simulink model "Parameter_Estimation_2020b"  (R2021a)
settings: Solver=ode2  StartTime=0.0  StopTime=9.999  FixedStep=0.001  RelTol=1e-3  EnableMultiTasking=on
StopFcn:
  | clc;
  | display('--------------------------------------------')
  | display('Running Least Squares Estimatation')
  | display('--------------------------------------------')
  | 
  | L = length (Least_Squares_Data.signals.values(:,1));
  | n = round (0.1*L);
  | m = round (0.9*L);
  | 
  | V = Least_Squares_Data.signals.values(n:m,1);
  | I = Least_Squares_Data.signals.values(n:m,2).*sign(V);
  | q_dot = Least_Squares_Data.signals.values(n:m,3);
  | sign_q_dot = Least_Squares_Data.signals.values(n:m,4);
  | I_dot = Least_Squares_Data.signals.values(n:m,5);
  | q_dbl_dot = Least_Squares_Data.signals.values(n:m,6);
  | K = ones (m-n,1);
  | 
  | A = [I q_dot sign_q_dot];
  | x = A\V;
  | 
  | display('Motor resistance (ohms)')
  | R = x(1)
  | display('Motor Speed constant (Vs/rad)')
  | Km = x(2)
  | 
  | B = [q_dbl_dot q_dot sign_q_dot];
  | tau = Km*I;
  | y = B\tau;
  | 
  | display('Motor inertia (kg m2)')
  | J = y(1)
  | display('Motor damping (Nm s/rad)')
  | B = y(2)
  | display('Coloumb torque constant (Nm)')
  | C = y(3)
  | display('--------------------------------------------')
undefined symbols (not defined in the file or in its folder): HIL
libraries: quarc_library x7
settings Model: SimulationMode=external  ExtModeTrigDuration=10000  Creator=mbohra  LastModifiedBy=user
settings SolverCC: AlgebraicLoopSolver=TrustRegion  PositivePriorityOrder=on
settings DataIOCC: SaveOutput=off  SignalLogging=off  DSMLogging=off  SaveTime=off  ReturnWorkspaceOutputs=off
settings DebuggingCC: SFMachineParentedDataDiag=warning  ArithmeticOperatorsInVariantConditions=warning
settings HardwareCC: ProdBitPerLong=64  ProdLargestAtomicInteger=LongLong  ProdLargestAtomicFloat=Double  ProdLongLongMode=on  ProdHWDeviceType=ARM Compatible->ARM 64-bit (LP64)
settings SFSimCC: CustomCodeUndefinedFunction=UseInterfaceOnly
settings RTWCC: Description=QUARC Linux Nvidia Target (QCar) Using Toolchain  SystemTargetFile=quarc_linux_nvidia.tlc  TemplateMakefile=quarc_default_tmf  Toolchain=QUARC linux_nvidia | gmake (64-bit Windows)  BuildConfiguration=Faster Runs
settings STFCustomTargetCC: TargetLangStandard=C99 (ISO)  ConcurrentExecutionCompliant=on  SystemTargetFile=quarc_linux_nvidia.tlc
settings GRTTargetCC: ParMdlRefBuildCompliant=off  CompOptLevelCompliant=off  CombineOutputUpdateFcns=off  MatFileLogging=off  CPPClassGenCompliant=off  GRTInterface=on  ExtMode=on  ExtModeMexFile=quarc_comm  ExtModeMexArgs='-w -d /tmp -uri %u', 'tcpip://192.168.1.9'

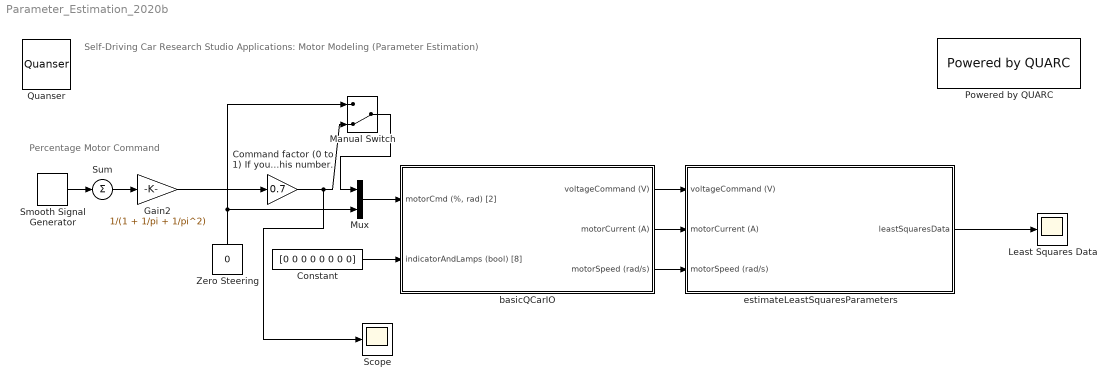
== system Parameter_Estimation_2020b ==
  note: Percentage Motor Command
  note: Self-Driving Car Research Studio
      | Applications: Motor Modeling (Parameter Estimation)
  "Command factor (0 to 1) If your room is small or the floor is slippery, reduce this number." : Gain  Gain=0.7
  Constant : Constant  Value=[0 0 0 0 0 0 0 0]
  Gain2 : Gain  Gain=1/(1 + 1/pi + 1/pi^2)
  Least Squares Data : Scope
  Manual Switch : ManualSwitch  CurrentSetting=0
  Mux : Mux  Inputs=2
  Powered by QUARC : quarc_library/Logos/Powered by QUARC
  Quanser : quarc_library/Logos/Quanser
  Scope : Scope
  Smooth Signal Generator : quarc_library/Sources/Signals/Smooth Signal Generator  signal_type=Sine  source=Internal (dialog parameters)  amplitude=[1 1/pi 1/pi^2]  frequency=[0.50 2 10]  initial_phase=0  sample_time=qc_get_step_size  output_cos=off
      settings: SourceProductName=QUARC Targets
  Sum : Sum  Inputs=1
  Zero Steering : Constant  Value=0
  basicQCarIO : Subsystem
  estimateLeastSquaresParameters : Subsystem
  wires:
  Constant/1 -> basicQCarIO/2(indicatorAndLamps (bool) [8])
  Smooth Signal Generator/1 -> Sum/1
  Sum/1 -> Gain2/1
  Mux/1 -> basicQCarIO/1("motorCmd (%, rad) [2]")
  Zero Steering/1 -> Mux/2, Manual Switch/1
  basicQCarIO/1(voltageCommand (V)) -> estimateLeastSquaresParameters/1("voltageCommand (V) ")
  basicQCarIO/2(motorCurrent (A)) -> estimateLeastSquaresParameters/2(motorCurrent (A))
  basicQCarIO/3(motorSpeed (rad/s)) -> estimateLeastSquaresParameters/3(motorSpeed (rad/s))
  estimateLeastSquaresParameters/1(leastSquaresData) -> Least Squares Data/1
  Gain2/1 -> "Command factor (0 to 1) If your room is small or the floor is slippery, reduce this number."/1
  "Command factor (0 to 1) If your room is small or the floor is slippery, reduce this number."/1 -> Scope/1, Manual Switch/2
  Manual Switch/1 -> Mux/1

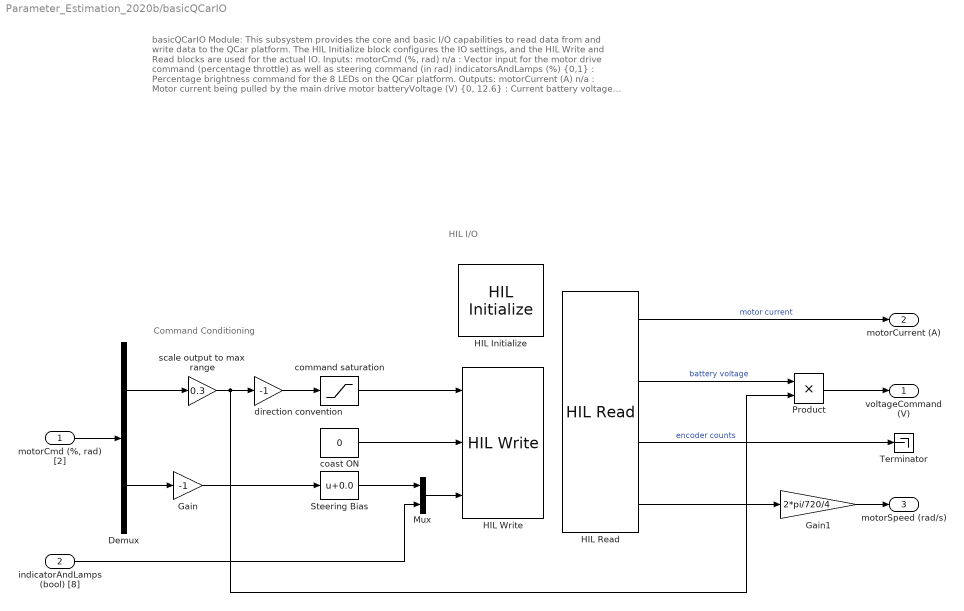
== system Parameter_Estimation_2020b/basicQCarIO ==
  note: basicQCarIO Module:
      |
      | This subsystem provides the core and basic I/O capabilities to read data from and write data to the QCar platform. The HIL Initialize block configures the IO settings, and the HIL Write and Read blocks are used for the actual IO.
      |
      | Inputs:
      | motorCmd (%, rad) n/a : Vector input for the motor drive command (percentage throttle) as well as steering command (in rad)
      | indicatorsAndLamps (%) {0,1} : Percentage brightness command for the 8 LEDs on the QCar platform.
      |
      | Outputs:
      | motorCurrent (A) n/a : Motor current being pulled by the main drive motor
      | batteryVoltage (V) {0, 12.6} : Current battery voltage reading
      | motorSpeed (counts/s) n/a : Drive motor speed measured using an encoder (do not confuse with wheel speed as this measurement is at the drive shaft)
  note: Command Conditioning
  note: HIL I/O
  "motorCmd (%, rad) [2]" : Inport
  indicatorAndLamps (bool) [8] : Inport  Port=2
  Demux : Demux  Outputs=2
  Gain : Gain  Gain=-1
  Gain1 : Gain  Gain=2*pi/720/4
  HIL Initialize : quarc_library/Data Acquisition/Generic/Configuration/HIL Initialize  object_name=HIL-1  board_type=qcar  board_number=0  board_options=gyro_fs=250;gyro_rate=64;accel_fs=2;accel_rate=62.5;mag_rate=20;mag_xy=47;mag_z=83;enc1_dir=0;enc2_dir=0;enc3_dir=0;enc4_dir=0;pwm1_dshot=0;pwm2_dshot=0;pwm3_dshot=0;pwm4_dshot=0;pwm5_dshot=0;pwm6_dshot=0;pwm7_dshot=0;steer_bias=0.05;motor_limit=0.3;  exclusive=off  active=on  hardware_clocks=[]  clock_modes=[]  initial_clock_frequencies=[]  set_clock_params_at_start=off  set_clock_params_at_switch_in=off  set_clock_frequencies_at_start=off  set_clock_frequencies_at_switch_in=off  analog_input_channels=[0:6]  analog_input_configurations=[]  analog_input_maximums=[3.3]  analog_input_minimums=[0]  set_analog_input_params_at_start=off  set_analog_input_params_at_switch_in=off  analog_output_channels=[]  analog_output_maximums=[]  analog_output_minimums=[]  initial_analog_outputs=[]  final_analog_outputs=[]  watchdog_analog_outputs=[]  set_analog_output_params_at_start=off  set_analog_output_params_at_switch_in=off  set_analog_outputs_at_start=off  set_analog_outputs_at_switch_in=off  set_analog_outputs_at_terminate=off  set_analog_outputs_at_switch_out=off  set_analog_outputs_on_watchdog=off  digital_input_channels=[24:43]  digital_output_channels=[40]  digital_output_configuration=[]  initial_digital_outputs=[0]  final_digital_outputs=[1]  watchdog_digital_outputs=[]  set_digital_output_params_at_start=off  set_digital_output_params_at_switch_in=off  set_digital_outputs_at_start=on  set_digital_outputs_at_switch_in=off  set_digital_outputs_at_terminate=on  set_digital_outputs_at_switch_out=off  set_digital_outputs_on_watchdog=off  encoder_channels=[0:4]  quadrature=[4 4]  encoder_filter_frequency=100e6/1  initial_encoder_counts=[0]  set_encoder_params_at_start=on  set_encoder_params_at_switch_in=off  set_encoder_counts_at_start=on  set_encoder_counts_at_switch_in=off  pwm_channels=[0:7]  pwm_modes=[0 0]  pwm_frequency=150e6/4096  pwm_configuration=[0]  pwm_alignment=[0]  pwm_polarity=[1]  pwm_leading_deadband=[]  pwm_trailing_deadband=[]  initial_pwm_outputs=[0]  final_pwm_outputs=[0]  watchdog_pwm_outputs=[0]  set_pwm_params_at_start=on  set_pwm_params_at_switch_in=off  set_pwm_outputs_at_start=on  set_pwm_outputs_at_switch_in=off  set_pwm_outputs_at_terminate=on  set_pwm_outputs_at_switch_out=off  set_pwm_outputs_on_watchdog=off  other_output_channels=[1000, 11000:11011]  initial_other_outputs=[0]  final_other_outputs=[0]  watchdog_other_outputs=[]  set_other_outputs_at_start=on  set_other_outputs_at_switch_in=off  set_other_outputs_at_terminate=on  set_other_outputs_at_switch_out=off  set_other_outputs_on_watchdog=off
  HIL Read : quarc_library/Data Acquisition/Generic/Immediate I//O/HIL Read  object_name=HIL-1  analog_channels=[5:6]  encoder_channels=[0]  digital_channels=[]  other_channels=[14000]  sample_time=qc_get_step_size  active=on  vector_output=off  data_type_mode=Inherit via back propagation  encoder_data_type=double  digital_data_type=boolean
  HIL Write : quarc_library/Data Acquisition/Generic/Immediate I//O/HIL Write  object_name=HIL-1  analog_channels=[]  pwm_channels=[0]  digital_channels=[40]  other_channels=[1000 11008:11011 11000:11003]  sample_time=-1  active=off  vector_input=on
  Mux : Mux  Inputs=2
  Product : Product
  Steering Bias : Bias  Bias=0.0
  Terminator : Terminator
  coast ON : Constant  Value=0
  command saturation : Saturate  UpperLimit=0.30  LowerLimit=-0.30
  direction convention : Gain  Gain=-1
  scale output to max range : Gain  Gain=0.3
  voltageCommand (V) : Outport  VectorParamsAs1DForOutWhenUnconnected=off
  motorCurrent (A) : Outport  Port=2  VectorParamsAs1DForOutWhenUnconnected=off
  motorSpeed (rad/s) : Outport  Port=3  VectorParamsAs1DForOutWhenUnconnected=off
  wires:
  Demux/2 -> Gain/1
  "motorCmd (%, rad) [2]"/1 -> Demux/1
  command saturation/1 -> HIL Write/1
  coast ON/1 -> HIL Write/2
  indicatorAndLamps (bool) [8]/1 -> Mux/2
  Steering Bias/1 -> Mux/1
  Mux/1 -> HIL Write/3
  Demux/1 -> scale output to max range/1
  Gain/1 -> Steering Bias/1
  HIL Read/1 -> motorCurrent (A)/1  "motor current"
  HIL Read/2 -> Product/1  "battery voltage"
  Gain1/1 -> motorSpeed (rad/s)/1
  Product/1 -> voltageCommand (V)/1
  direction convention/1 -> command saturation/1
  HIL Read/4 -> Gain1/1
  HIL Read/3 -> Terminator/1  "encoder counts"
  scale output to max range/1 -> Product/2, direction convention/1

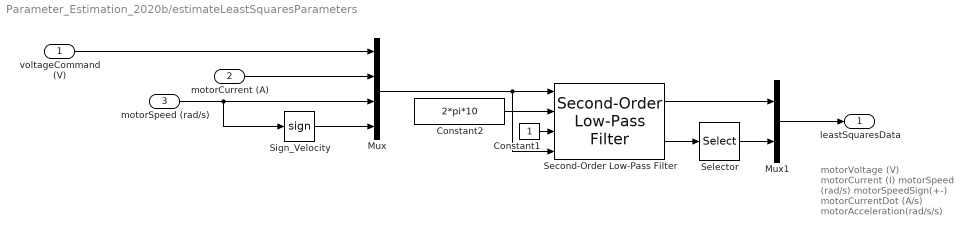
== system Parameter_Estimation_2020b/estimateLeastSquaresParameters ==
  note: motorVoltage (V)
      | motorCurrent (I)
      | motorSpeed (rad/s)
      | motorSpeedSign(+-)
      | motorCurrentDot (A/s)
      | motorAcceleration(rad/s/s)
  "voltageCommand (V) " : Inport
  motorCurrent (A) : Inport  Port=2
  motorSpeed (rad/s) : Inport  Port=3
  Constant1 : Constant
  Constant2 : Constant  Value=2*pi*10
  Mux : Mux
  Mux1 : Mux  Inputs=2
  Second-Order Low-Pass Filter : quarc_library/Continuous/Second-Order Low-Pass Filter  params_source=External (input ports)  input_width=1  input_zeta=1  input_init=0
  Selector : Selector  InputPortWidth=4  IndexOptions=Index vector (dialog)  Indices=2:3  OutputSizes=1
  Sign_Velocity : Signum
  leastSquaresData : Outport  VectorParamsAs1DForOutWhenUnconnected=off
  wires:
  Selector/1 -> Mux1/2
  Second-Order Low-Pass Filter/1 -> Mux1/1
  Second-Order Low-Pass Filter/2 -> Selector/1
  Constant1/1 -> Second-Order Low-Pass Filter/3
  Constant2/1 -> Second-Order Low-Pass Filter/2
  Mux/1 -> Second-Order Low-Pass Filter/4, Second-Order Low-Pass Filter/1
  "voltageCommand (V) "/1 -> Mux/1
  motorSpeed (rad/s)/1 -> Sign_Velocity/1, Mux/3
  Mux1/1 -> leastSquaresData/1
  Sign_Velocity/1 -> Mux/4
  motorCurrent (A)/1 -> Mux/2
